simulink model "ksi_ver"  (R2019a)
settings: Solver=VariableStepAuto  StartTime=0.0  StopTime=(nSamp-1)*Ts  RelTol=1e-3
InitFcn:
  | block_verScript;
StopFcn:
  | ksiOut = out.ksi_verOut.signals.values(:, 1:FFT_size);
  | hwOut = out.hw_verOut.signals.values(:, 1:FFT_size);
  | 
  | figure();
  | subplot(211);
  | stem(1:FFT_size, ksiOut(1,:)); xlabel('Samples'); title('ksi Output - Frame 1');
  | subplot(212);
  | stem(1:FFT_size, hwOut(1,:)); xlabel('Samples'); title('hw Output - Frame 1');
values from neighbouring files (symbols this model uses):
  FFT_size = 64    [FIR_filterTestm.m]    (also in JMAP_INIT.m; blockVerification.m; block_verScript.m; ksi_verScript.m)
  ksiMin = 0.0032*ones(FFT_size, 1)    [JMAP_INIT.m]    (also in block_verScript.m = 0.0032; ksi_verScript.m = 0.0032)
  Ts = 1/Fs    (= 2.08333333333e-05)    [FIR_filterTestm.m]    (also in JMAP_INIT.m; blockVerification.m; block_verScript.m; ksi_verScript.m)
libraries: simulink x2
settings Model: Creator=Showi  LastModifiedBy=Showi

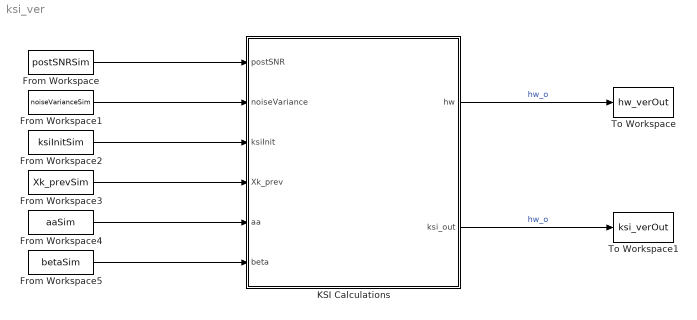
== system ksi_ver ==
  From Workspace : FromWorkspace  VariableName=postSNRSim  SampleTime=Ts
  From Workspace1 : FromWorkspace  VariableName=noiseVarianceSim  SampleTime=Ts
  From Workspace2 : FromWorkspace  VariableName=ksiInitSim  SampleTime=Ts
  From Workspace3 : FromWorkspace  VariableName=Xk_prevSim  SampleTime=Ts
  From Workspace4 : FromWorkspace  VariableName=aaSim  SampleTime=Ts
  From Workspace5 : FromWorkspace  VariableName=betaSim  SampleTime=Ts
  KSI Calculations : Subsystem
  To Workspace : ToWorkspace  VariableName=hw_verOut  SaveFormat=Structure With Time  SampleTime=-1
  To Workspace1 : ToWorkspace  VariableName=ksi_verOut  SaveFormat=Structure With Time  SampleTime=-1
  wires:
  From Workspace/1 -> KSI Calculations/1(postSNR)
  From Workspace1/1 -> KSI Calculations/2(noiseVariance)
  From Workspace2/1 -> KSI Calculations/3(ksiInit)
  From Workspace3/1 -> KSI Calculations/4(Xk_prev)
  From Workspace4/1 -> KSI Calculations/5(aa)
  From Workspace5/1 -> KSI Calculations/6(beta)
  KSI Calculations/1(hw) -> To Workspace/1  "hw_o"
  KSI Calculations/2(ksi_out) -> To Workspace1/1  "hw_o"

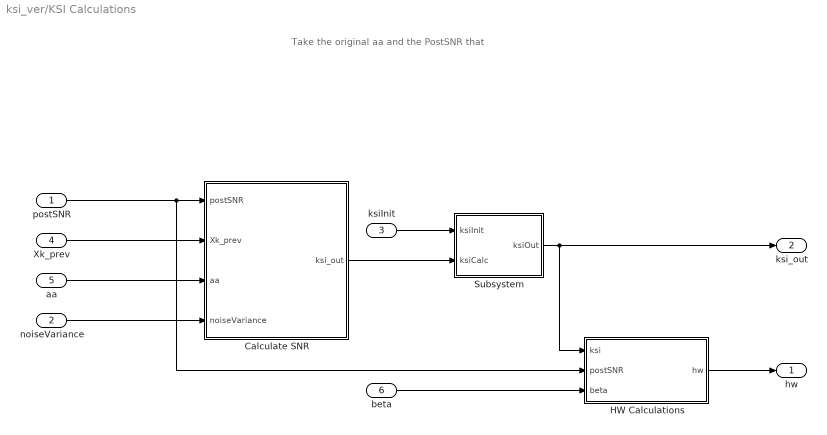
== system ksi_ver/KSI Calculations ==
  note: Take the original aa and the PostSNR that
  postSNR : Inport
  noiseVariance : Inport  Port=2
  ksiInit : Inport  Port=3
  Xk_prev : Inport  Port=4
  aa : Inport  Port=5
  beta : Inport  Port=6
  Calculate SNR : Subsystem
  HW Calculations : Subsystem
  Subsystem : Subsystem
  hw : Outport
  ksi_out : Outport  Port=2
  wires:
  noiseVariance/1 -> Calculate SNR/4(noiseVariance)
  beta/1 -> HW Calculations/3(beta)
  postSNR/1 -> HW Calculations/2(postSNR), Calculate SNR/1(postSNR)
  Xk_prev/1 -> Calculate SNR/2(Xk_prev)
  aa/1 -> Calculate SNR/3(aa)
  HW Calculations/1(hw) -> hw/1
  Subsystem/1(ksiOut) -> HW Calculations/1(ksi), ksi_out/1
  ksiInit/1 -> Subsystem/1(ksiInit)
  Calculate SNR/1(ksi_out) -> Subsystem/2(ksiCalc)

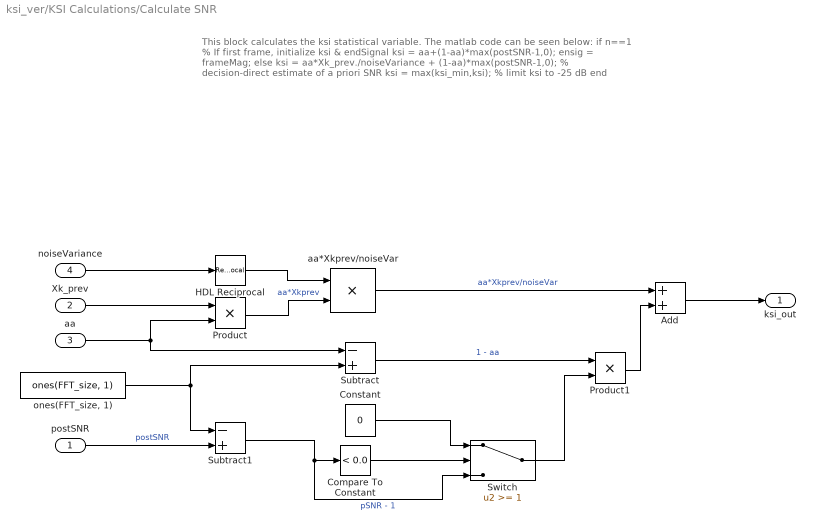
== system ksi_ver/KSI Calculations/Calculate SNR ==
  note: This block calculates the ksi statistical variable.
      |
      | The matlab code can be seen below:
      |
      |     if n==1 % If first frame, initialize ksi & endSignal
      |         ksi = aa+(1-aa)*max(postSNR-1,0);
      |         ensig = frameMag;
      |     else
      |         ksi = aa*Xk_prev./noiseVariance + (1-aa)*max(postSNR-1,0);
      |         % decision-direct estimate of a priori SNR
      |         ksi = max(ksi_min,ksi);  % limit ksi to -25 dB
      |     end
  postSNR : Inport
  Xk_prev : Inport  Port=2
  aa : Inport  Port=3
  noiseVariance : Inport  Port=4
  Add : Sum
  Compare To Constant : simulink/Logic and Bit Operations/Compare To Constant  relop=<  const=0.0  OutDataTypeStr=boolean
  Constant : Constant  Value=0  SampleTime=-1
  HDL Reciprocal : Reciprocal
  Product : Product
  Product1 : Product
  Subtract : Sum  Inputs=-+
  Subtract1 : Sum  Inputs=-+
  Switch : Switch  Threshold=1
  aa*Xkprev/noiseVar : Product  Inputs=**  SaturateOnIntegerOverflow=on  RndMeth=Zero
  "ones(FFT_size, 1)" : Constant  Value=ones(FFT_size, 1)  SampleTime=-1
  ksi_out : Outport
  wires:
  Add/1 -> ksi_out/1
  Xk_prev/1 -> Product/1
  aa/1 -> Subtract/1, Product/2
  Product/1 -> aa*Xkprev/noiseVar/2  "aa*Xkprev"
  noiseVariance/1 -> HDL Reciprocal/1
  "ones(FFT_size, 1)"/1 -> Subtract/2, Subtract1/1
  postSNR/1 -> Subtract1/2  "postSNR"
  Subtract/1 -> Product1/1  "1 - aa"
  Subtract1/1 -> Switch/3, Compare To Constant/1  "pSNR - 1"
  Product1/1 -> Add/2
  aa*Xkprev/noiseVar/1 -> Add/1  "aa*Xkprev/noiseVar"
  HDL Reciprocal/1 -> aa*Xkprev/noiseVar/1
  Compare To Constant/1 -> Switch/2
  Constant/1 -> Switch/1
  Switch/1 -> Product1/2

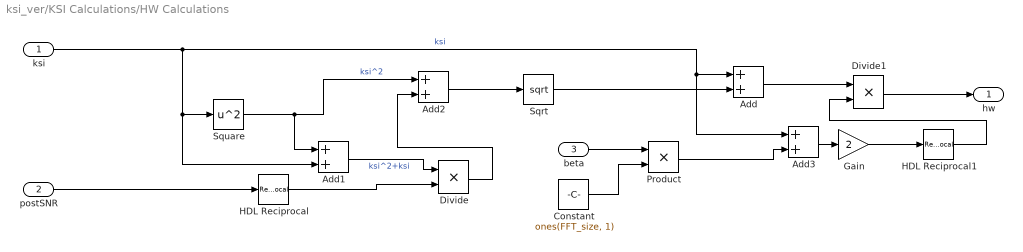
== system ksi_ver/KSI Calculations/HW Calculations ==
  ksi : Inport
  postSNR : Inport  Port=2
  beta : Inport  Port=3
  Add{,1..3} (4 alike) : Sum
  Constant : Constant  Value=ones(FFT_size, 1)  SampleTime=Ts
  Divide : Product  Inputs=**  SaturateOnIntegerOverflow=on  RndMeth=Zero
  Divide1 : Product  Inputs=**  SaturateOnIntegerOverflow=on  RndMeth=Zero
  Gain : Gain  Gain=2
  HDL Reciprocal : Reciprocal
  HDL Reciprocal1 : Reciprocal
  Product : Product
  Sqrt : Sqrt  SaturateOnIntegerOverflow=on
  Square : Math  Operator=square  RndMeth=Zero  SaturateOnIntegerOverflow=on
  hw : Outport
  wires:
  ksi/1 -> Square/1, Add1/2, Add3/1, Add/1  "ksi"
  Square/1 -> Add2/1, Add1/1  "ksi^2"
  Sqrt/1 -> Add/2
  Add2/1 -> Sqrt/1
  beta/1 -> Product/1
  Add3/1 -> Gain/1
  Divide1/1 -> hw/1
  Add/1 -> Divide1/1
  Gain/1 -> HDL Reciprocal1/1
  postSNR/1 -> HDL Reciprocal/1
  Add1/1 -> Divide/1  "ksi^2+ksi"
  Divide/1 -> Add2/2
  Constant/1 -> Product/2
  Product/1 -> Add3/2
  HDL Reciprocal/1 -> Divide/2
  HDL Reciprocal1/1 -> Divide1/2

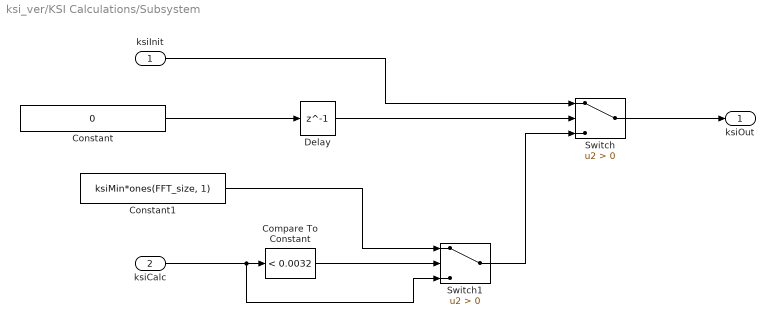
== system ksi_ver/KSI Calculations/Subsystem ==
  ksiInit : Inport
  ksiCalc : Inport  Port=2
  Compare To Constant : simulink/Logic and Bit Operations/Compare To Constant  relop=<  const=0.0032  OutDataTypeStr=boolean
  Constant : Constant  Value=0  SampleTime=-1
  Constant1 : Constant  Value=ksiMin*ones(FFT_size, 1)  SampleTime=-1
  Delay : Delay  DelayLength=1  InitialCondition=1
  Switch : Switch  Criteria=u2 > Threshold
  Switch1 : Switch  Criteria=u2 > Threshold
  ksiOut : Outport
  wires:
  Constant/1 -> Delay/1
  Switch1/1 -> Switch/3
  Constant1/1 -> Switch1/1
  ksiInit/1 -> Switch/1
  ksiCalc/1 -> Switch1/3, Compare To Constant/1
  Compare To Constant/1 -> Switch1/2
  Delay/1 -> Switch/2
  Switch/1 -> ksiOut/1
